simulink model "test_fmu_v3"  (R2022a)
settings: Solver=FixedStepAuto  StartTime=0.0  StopTime=10.0  RelTol=1e-3
undefined symbols (not defined in the file or in its folder): FMIKit
libraries: spspowerguiLib x1
settings Model: Creator=lordx  LastModifiedBy=lordx
settings SFSimCC: SimUserSources="\"F:\\GitHubRepos\\Test_FMU_2\\test_fmu_v1\\sources\\test_fmu_v1.c\" \"F:\\GitHubRepos\\Test_FMU_2\\test_fmu_v1\\sources\\test_fmu_v1_data.c\" \"F:\\GitHubRepos\\Test_FMU_2\\test_fmu_v1\\sources\\RTWCG_FMU_util.c\" \"F:\\GitHubRepos\\Test_FMU_2\\test_fmu_v1\\sources\\test_fmu_v1_fmu.c\""  SimUserIncludeDirs="\"D:\\Program Files\\Matlab\\rtw\\c\\FMIKit-Simulink-3.0\" \"D:\\Program Files\\Matlab\\rtw\\c\\FMIKit-Simulink-3.0\\include\" \"F:\\GitHubRepos\\Test_FMU_2\\test_fmu_v1\\sources\""
settings RTWCC: Description=FMU based on GRT (Functional Mock-up Unit)  SystemTargetFile=grtfmi.tlc  GenerateMakefile=off  TemplateMakefile=none  GenerateReport=on  RetainRTWFile=on  CustomInclude="\"D:\\Program Files\\Matlab\\rtw\\c\\FMIKit-Simulink-3.0\" \"D:\\Program Files\\Matlab\\rtw\\c\\FMIKit-Simulink-3.0\\include\" \"F:\\GitHubRepos\\Test_FMU_2\\test_fmu_v1\\sources\""  CustomSource="\"F:\\GitHubRepos\\Test_FMU_2\\test_fmu_v1\\sources\\test_fmu_v1.c\" \"F:\\GitHubRepos\\Test_FMU_2\\test_fmu_v1\\sources\\test_fmu_v1_data.c\" \"F:\\GitHubRepos\\Test_FMU_2\\test_fmu_v1\\sources\\RTWCG_FMU_util.c\" \"F:\\GitHubRepos\\Test_FMU_2\\test_fmu_v1\\sources\\test_fmu_v1_fmu.c\""
settings CodeAppCC: ForceParamTrailComments=on  StateflowObjectComments=on  MATLABSourceComments=on
settings STFCustomTargetCC: TargetLangStandard=C99 (ISO)  CombineOutputUpdateFcns=on  GRTInterface=off  OptimizeReductions=on  SystemTargetFile=grtfmi.tlc
settings GRTTargetCC: ParMdlRefBuildCompliant=off  CompOptLevelCompliant=off  ConcurrentExecutionCompliant=off  MatFileLogging=off  CPPClassGenCompliant=off  UseToolchainInfoCompliant=off  OptimizeReductions=on  RTWCAPISignals=on  RTWCAPIParams=on  RTWCAPIStates=on  RTWCAPIRootIO=on

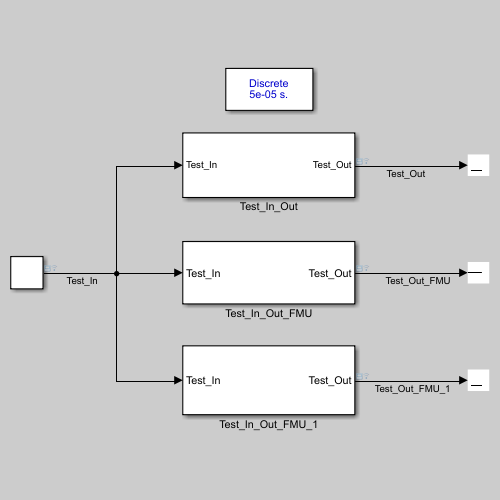
[thumbnail: Simulink's stored preview of the top-level diagram]
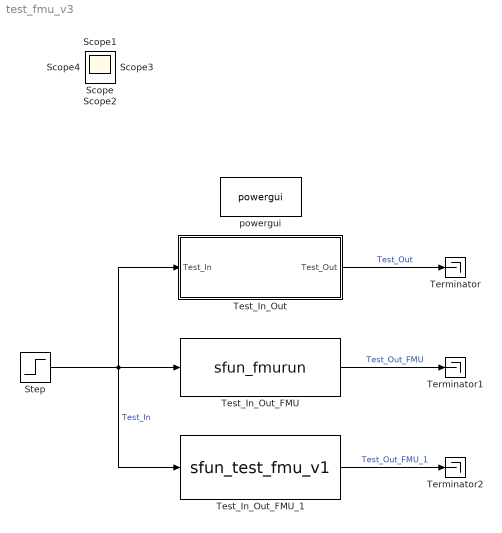
== system test_fmu_v3 ==
  Step : Step  Time=0  SampleTime=0
  Terminator : Terminator
  Terminator1 : Terminator
  Terminator2 : Terminator
  Test_In_Out : Subsystem
  Test_In_Out_FMU : S-Function  LoadFcn=FMIKit.setSFunctionParameters(gcb)  FunctionName=sfun_fmurun  Parameters=3.0 1 '{215efcaa-77a9-424c-8dc7-1b7a98b1376d}' 'test_fmu' FMIKit.getUnzipDirectory(gcb) 1 1 0 'test_fmu_v3_FMU.txt' 0.01 -1 0 0 0 0 [1] [0] [2] [2] [1] [2] [3] 0 0 2 1 Parameters_Gain_Gain  SFunctionDeploymentMode=off  EnableBusSupport=off  mask{Parameters_Gain_Gain=100}
      mask prompts: Parameters_Gain_Gain "Parameters.Gain_Gain"
      settings: DeleteFcn=FMIKit.closeBlockDialog(gcbh)  ModelCloseFcn=FMIKit.closeBlockDialog(gcbh)  DestroyFcn=FMIKit.closeBlockDialog(gcbh)  OpenFcn=FMIKit.showBlockDialog(gcbh);  CloseFcn=FMIKit.closeBlockDialog(gcbh)  ParentCloseFcn=FMIKit.closeBlockDialog(gcbh)
      mask Help: eval('FMIKit.showBlockDialogHelp();')
      mask Display:
      | port_label('input', 1, 'Test_In');
      | port_label('output', 1, 'Test_Out');
  Test_In_Out_FMU_1 : S-Function  LoadFcn=FMIKit.setSFunctionParameters(gcb)  FunctionName=sfun_test_fmu_v1  Parameters=2.0 1 '{7390c40e-2681-d7d3-36c9-f59522b69178}' 'test_fmu_v1' FMIKit.getUnzipDirectory(gcb) 1 1 0 'test_fmu_v3_FMU.txt' 0 -1 0 0 0 0 [1] [0] [2] [0] [1] [2] [1]  SFunctionDeploymentMode=off  EnableBusSupport=off
      settings: DeleteFcn=FMIKit.closeBlockDialog(gcbh)  ModelCloseFcn=FMIKit.closeBlockDialog(gcbh)  DestroyFcn=FMIKit.closeBlockDialog(gcbh)  OpenFcn=FMIKit.showBlockDialog(gcbh);  CloseFcn=FMIKit.closeBlockDialog(gcbh)  ParentCloseFcn=FMIKit.closeBlockDialog(gcbh)
      mask Help: eval('FMIKit.showBlockDialogHelp();')
      mask Display:
      | port_label('input', 1, 'Test_In');
      | port_label('output', 1, 'Test_Out');
  powergui : spspowerguiLib/powergui  Priority=1  SimulationMode=Discrete  SampleTime=50e-6  frequency=60  Iterations=50  frequencyindice=60  Pbase=100e6  ErrMax=1e-4  UnitsV=kV  UnitsW=MW  buscounter=0  FunctionMessages=off  echomessages=off  EnableUseOfTLC=off  CurrentSourceSwitches=off  DisableSnubberDevices=off  DisableRonSwitches=off  DisableVfSwitches=off  DisplayEquations=off  AutomaticDiscreteSolvers=off  SolverType=Tustin/Backward Euler (TBE)  Interpol=off  ExternalGateDelay=off  methode=off  Ts=100  x0status=blocks  SPID=on  SwTol=0  HookPort=off  NonlinearTolerance=1e-4  nMaxIteration=100  ContinueOnMaxIteration=off  RestoreLinks=warning  ResistiveCurrentMeasurement=off  Frange=[0:2:500]  Ylog=off  Xlog=on  ShowGrid=off  save=off  variable=ZData  structure=0  ZoomFFT=off  StartTime=0.0  cycles=1  DisplayStyle=1  fundamental=60  FreqAxis=off  MaxFrequency=1000  frequencyindicesteady=1  RmsSteady=1  display=off
  Scope{,1..4} (5 alike) : Scope
  wires:
  Step/1 -> Test_In_Out/1(Test_In), Test_In_Out_FMU_1/1, Test_In_Out_FMU/1  "Test_In"
  Test_In_Out/1(Test_Out) -> Terminator/1  "Test_Out"
  Test_In_Out_FMU/1 -> Terminator1/1  "Test_Out_FMU"
  Test_In_Out_FMU_1/1 -> Terminator2/1  "Test_Out_FMU_1"

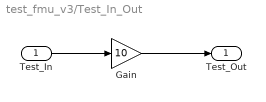
== system test_fmu_v3/Test_In_Out ==
  Test_In : Inport
  Gain : Gain  Gain=10
  Test_Out : Outport
  wires:
  Test_In/1 -> Gain/1
  Gain/1 -> Test_Out/1
